simulink model "sim_PI_controller"  (R2018a)
settings: Solver=ode45  StartTime=0.0  StopTime=2  RelTol=1e-3
model workspace: external: MAT-File workspace_simulink_params.mat (data not in the file)
values from neighbouring files (symbols this model uses):
  denominator = [1 342.893035076 21085141.153]    [workspace_simulink_params.mat]
  disturbance_amplitude = 0.5    [plant_estimation_and_controller_design.m]
  disturbance_frequency = 10    [plant_estimation_and_controller_design.m]
  disturbance_offset = 0.5    [plant_estimation_and_controller_design.m]
  disturbance_phase = 0    [plant_estimation_and_controller_design.m]
  KI = KP/TN    [plant_estimation_and_controller_design.m]
  KP = 1.2*Tg/(Ks*Tv)    [plant_estimation_and_controller_design.m]
  numerator = [0 73.7642635112 10477310.7512]    [workspace_simulink_params.mat]
  step_gain = 1    [plant_estimation_and_controller_design.m]
  step_time = 1    [plant_estimation_and_controller_design.m]    (also in workspace_simulink_params.mat)
settings Model: Creator=Patrick  LastModifiedBy=Gsoels

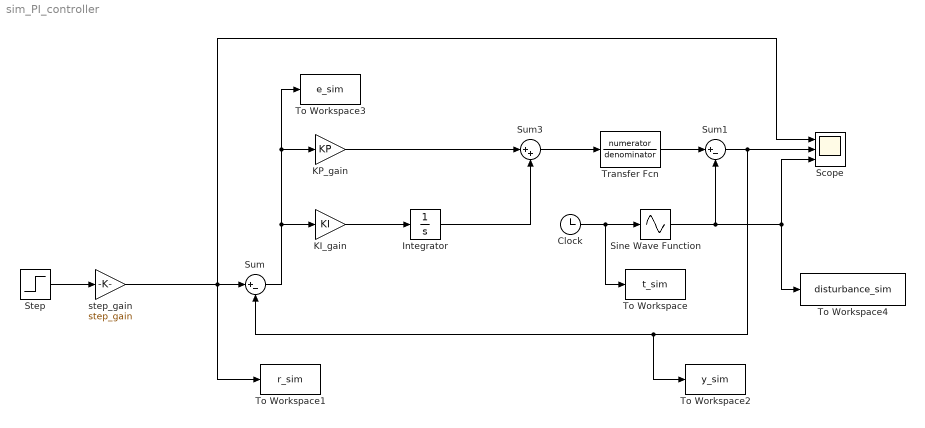
== system sim_PI_controller ==
  Clock : Clock
  Integrator : Integrator
  KI_gain : Gain  Gain=KI
  KP_gain : Gain  Gain=KP
  Scope : Scope  NumInputPorts=3
  Sine Wave Function : Sin  TimeSource=Use external signal  Amplitude=disturbance_amplitude  Bias=disturbance_offset  Frequency=disturbance_frequency  Phase=disturbance_phase  SampleTime=0
  Step : Step  Time=step_time  SampleTime=0
  Sum : Sum  Inputs=|+-
  Sum1 : Sum  Inputs=|+-
  Sum3 : Sum  Inputs=|++
  To Workspace : ToWorkspace  VariableName=t_sim  SampleTime=-1
  To Workspace1 : ToWorkspace  VariableName=r_sim  SampleTime=-1
  To Workspace2 : ToWorkspace  VariableName=y_sim  SampleTime=-1
  To Workspace3 : ToWorkspace  VariableName=e_sim  SampleTime=-1
  To Workspace4 : ToWorkspace  VariableName=disturbance_sim  SampleTime=-1
  Transfer Fcn : TransferFcn  Numerator=numerator  Denominator=denominator
  step_gain : Gain  Gain=step_gain
  wires:
  Step/1 -> step_gain/1
  Transfer Fcn/1 -> Sum1/1
  Sine Wave Function/1 -> To Workspace4/1, Scope/3, Sum1/2
  Sum1/1 -> To Workspace2/1, Sum/2, Scope/2
  KI_gain/1 -> Integrator/1
  Sum/1 -> KP_gain/1, To Workspace3/1, KI_gain/1
  Integrator/1 -> Sum3/2
  KP_gain/1 -> Sum3/1
  Sum3/1 -> Transfer Fcn/1
  Clock/1 -> Sine Wave Function/1, To Workspace/1
  step_gain/1 -> To Workspace1/1, Scope/1, Sum/1
